simulink model "xy_graph"  (R2022a)
settings: Solver=VariableStepAuto  StartTime=0.0  StopTime=20  RelTol=1e-3
settings Model: Creator=Home  LastModifiedBy=Home

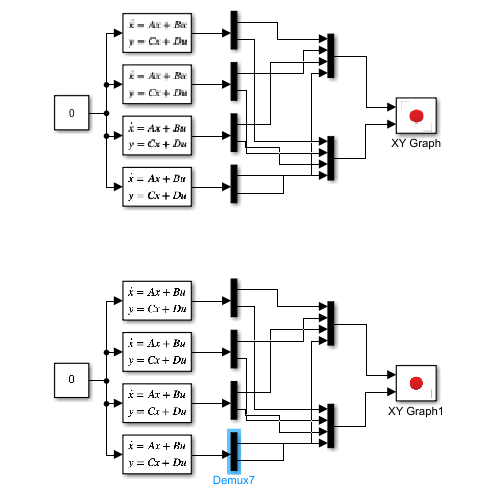
[thumbnail: Simulink's stored preview of the top-level diagram]
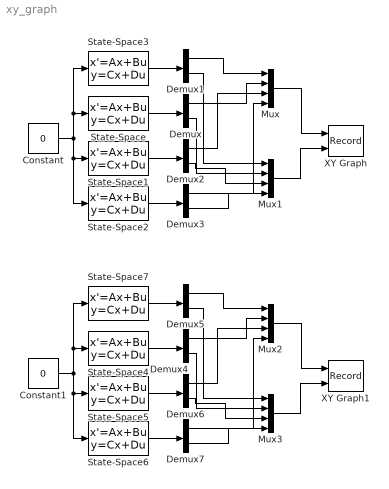
== system xy_graph ==
  Constant : Constant  Value=0
  Constant1 : Constant  Value=0
  Demux{,1..7} (8 alike) : Demux  Outputs=2
  Mux{,1..3} (4 alike) : Mux
  State-Space : StateSpace  A=[0 1; -2 1]  B=[0; 0]  C=eye(2)  D=[0; 0]  InitialCondition=[1 -1]
  State-Space1 : StateSpace  A=[0 1; -2 1]  B=[0; 0]  C=eye(2)  D=[0; 0]  InitialCondition=[-1 1]  ParameterTunability=Unconstrained
  State-Space2 : StateSpace  A=[0 1; -2 1]  B=[0; 0]  C=eye(2)  D=[0; 0]  InitialCondition=[-1 -1]  ParameterTunability=Unconstrained
  State-Space3 : StateSpace  A=[0 1; -2 1]  B=[0; 0]  C=eye(2)  D=[0; 0]  InitialCondition=[1 1]  ParameterTunability=Unconstrained
  State-Space4 : StateSpace  A=[-3 2; 1 -4]  B=[0; 0]  C=eye(2)  D=[0; 0]  InitialCondition=[500 -1000]
  State-Space5 : StateSpace  A=[-3 2; 1 -4]  B=[0; 0]  C=eye(2)  D=[0; 0]  InitialCondition=[-500 1000]  ParameterTunability=Unconstrained
  State-Space6 : StateSpace  A=[-3 2; 1 -4]  B=[0; 0]  C=eye(2)  D=[0; 0]  InitialCondition=[-500 -1000]  ParameterTunability=Unconstrained
  State-Space7 : StateSpace  A=[-3 2; 1 -4]  B=[0; 0]  C=eye(2)  D=[0; 0]  InitialCondition=[500 1000]  ParameterTunability=Unconstrained
  XY Graph : Record  FileSettingsInternal="{\"entries\":[{\"content\":{\"excelSettings\":{\"content\":{},\"type\":\"Streamout.ExcelSettings\"}},\"type\":\"Streamout.FileSettingStorage\",\"uuid\":\"1620cbbc-033e-4fe2-b11b-f0d51b19d3c6\"}],\"packageUris\":[\"http://schema.mathworks.com/mf0/streamout_blocks/R2020a\"],\"version\":\"1.0\"}"  Layout=[1 1]  SignalsInternal="{\"entries\":[{\"content\":{\"signals\":[{\"content\":{\"blockPath\":[\"xy_graph/XY Graph\"],\"channel\":[],\"dimensions\":[4],\"domain\":\"xy_graph/XY Graph\",\"hasChildren\":true,\"lineColor\":\"#edb120\",\"plots\":[],\"port\":1,\"sid\":[\"\"],\"signalID\":1160,\"signalName\":\"Mux\"},\"type\":\"RecordBlkView.Signal\",\"uuid\":\"24731fe2-5eeb-46e2-9522-8e4ef2046298\"},{\"content\":{\"blockPath\":[\"xy_graph/XY Graph\"],\"channel\":[1],\"dimensions\":[4],\"domain\":\"xy_graph/XY Graph\",\"lineColor\":\"#139fff\",\"parentID\":1160,\"plots\":[1],\"port\":1,\"sid\":[\"\"],\"signalID\":1161,\"signalName\":\"Mux\"},\"type\":\"RecordBlkView.Signal\",\"uuid\":\"67ca6b0b-c82a-407b-9284-4bd69131f7ea\"},{\"content\":{\"blockPath\":[\"xy_graph/XY Graph\"],\"channel\":[],\"dimensions\":[4],\"domain\":\"xy_graph/XY Graph\",\"hasChildren\":true,\"lineColor\":\"#77ac30\",\"plots\":[],\"port\":2,\"sid\":[\"\"],\"signalID\":1165,\"signalName\":\"Mux1\"},\"type\":\"RecordBlkView.Signal\",\"uuid\":\"273c0b79-0516-42a1-b449-bf05efc436ae\"},{\"content\":{\"blockPath\":[\"xy_graph/XY Graph\"],\"channel\":[1],\"dimensions\":[4],\"domain\":\"xy_graph/XY Graph\",\"lineColor\":\"#b746ff\",\"parentID\":1165,\"plots\":[1],\"port\":2,\"sid\":[\"\"],\"signalID\":1166,\"signalName\":\"Mux1\"},\"type\":\"RecordBlkView.Signal\",\"uuid\":\"56d8e83f-c520-44f4-8c35-4e371990f6b9\"},{\"content\":{\"blockPath\":[\"xy_graph/XY Graph\"],\"channel\":[2],\"dimensions\":[4],\"domain\":\"xy_graph/XY Graph\",\"lineColor\":\"#64d413\",\"parentID\":1160,\"plots\":[1],\"port\":1,\"sid\":[\"\"],\"signalID\":1180,\"signalName\":\"Mux\"},\"type\":\"RecordBlkView.Signal\",\"uuid\":\"527b7954-8048-4bae-9c72-ca187d897607\"},{\"content\":{\"blockPath\":[\"xy_graph/XY Graph\"],\"channel\":[3],\"dimensions\":[4],\"domain\":\"xy_graph/XY Graph\",\"lineColor\":\"#ff13a6\",\"parentID\":1160,\"plots\":[1],\"port\":1,\"sid\":[\"\"],\"signalID\":1181,\"signalName\":\"Mux\"},\"type\":\"RecordBlkView.Signal\",\"uuid\":\"88895bde-14ff-4988-9de3-88a08c4df239\"},{\"content\":{\"blockPath\":[\"xy_graph/XY Graph\"],\"channel\":[4],\"dimensions\":[4],\"domain\":\"xy_graph/XY Graph\",\"lineColor\":\"#fe330a\",\"parentID\":1160,\"plots\":[1],\"port\":1,\"sid\":[\"\"],\"signalID\":1182,\"signalName\":\"Mux\"},\"type\":\"RecordBlkView.Signal\",\"uuid\":\"b99bfa31-054d-46ce-93bd-0866448dc733\"},{\"content\":{\"blockPath\":[\"xy_graph/XY Graph\"],\"channel\":[2],\"dimensions\":[4],\"domain\":\"xy_graph/XY Graph\",\"lineColor\":\"#22b573\",\"parentID\":1165,\"plots\":[1],\"port\":2,\"sid\":[\"\"],\"signalID\":1183,\"signalName\":\"Mux1\"},\"type\":\"RecordBlkView.Signal\",\"uuid\":\"7f3c33f5-9ec2-4f34-b33e-4a0e5e9e8405\"},{\"content\":{\"blockPath\":[\"xy_graph/XY Graph\"],\"channel\":[3],\"dimensions\":[4],\"domain\":\"xy_graph/XY Graph\",\"lineColor\":\"#0072bd\",\"parentID\":1165,\"plots\":[1],\"port\":2,\"sid\":[\"\"],\"signalID\":1184,\"signalName\":\"Mux1\"},\"type\":\"RecordBlkView.Signal\",\"uuid\":\"b1473734-461a-42dd-896c-7caac445258d\"},{\"content\":{\"blockPath\":[\"xy_graph/XY Graph\"],\"channel\":[4],\"dimensions\":[4],\"domain\":\"xy_graph/XY Graph\",\"lineColor\":\"#d95319\",\"parentID\":1165,\"plots\":[1],\"port\":2,\"sid\":[\"\"],\"signalID\":1185,\"signalName\":\"Mux1\"},\"type\":\"RecordBlkView.Signal\",\"uuid\":\"044ac694-07e2-40e9-8c24-0635b6094aa9\"}]},\"type\":\"RecordBlkView.InputSignals\",\"uuid\":\"fb853018-507c-4a33-8839-1e66abb60dcd\"}],\"packageUris\":[\"http://schema.mathworks.com/mf0/streamout_blocks/R2020a\"],\"version\":\"1.0\"}"  VisualizationBindings="{\"xyplotplugin\":{\"info\":[{\"series\":[{\"bindingParametersList\":[{\"parameter\":\"X-Axis\",\"signalID\":1161,\"signalName\":\"Mux(1)\"},{\"parameter\":\"Y-Axis\",\"signalID\":1166,\"signalName\":\"Mux1(1)\"}],\"seriesID\":1003},{\"bindingParametersList\":[{\"parameter\":\"X-Axis\",\"signalID\":1180,\"signalName\":\"Mux(2)\"},{\"parameter\":\"Y-Axis\",\"signalID\":1183,\"signalName\":\"Mux1(2)\"}],\"seriesID\":908},{\"bindingParametersList\":[{\"parameter\":\"X-Axis\",\"signalID\":1181,\"signalName\":\"Mux(3)\"},{\"parameter\":\"Y-Axis\",\"signalID\":1184,\"signalName\":\"Mux1(3)\"}],\"seriesID\":917},{\"bindingParametersList\":[{\"parameter\":\"X-Axis\",\"signalID\":1182,\"signalName\":\"Mux(4)\"},{\"parameter\":\"Y-Axis\",\"signalID\":1185,\"signalName\":\"Mux1(4)\"}],\"seriesID\":762}],\"subplotID\":1}]}}"  CompatibilityTag=XY
  XY Graph1 : Record  FileSettingsInternal="{\"entries\":[{\"content\":{\"excelSettings\":{\"content\":{},\"type\":\"Streamout.ExcelSettings\"}},\"type\":\"Streamout.FileSettingStorage\",\"uuid\":\"14b4cfe2-687b-4cc5-8bba-4bb3a5f8f04c\"}],\"packageUris\":[\"http://schema.mathworks.com/mf0/streamout_blocks/R2020a\"],\"version\":\"1.0\"}"  Layout=[1 1]  SignalsInternal="{\"entries\":[{\"content\":{\"signals\":[{\"content\":{\"blockPath\":[\"xy_graph/XY Graph1\"],\"channel\":[],\"dimensions\":[4],\"domain\":\"xy_graph/XY Graph1\",\"hasChildren\":true,\"lineColor\":\"#a2142f\",\"plots\":[],\"port\":1,\"sid\":[\"\"],\"signalID\":1170,\"signalName\":\"Mux2\"},\"type\":\"RecordBlkView.Signal\",\"uuid\":\"c4bd5d30-0501-47c8-9430-780dbd134563\"},{\"content\":{\"blockPath\":[\"xy_graph/XY Graph1\"],\"channel\":[1],\"dimensions\":[4],\"domain\":\"xy_graph/XY Graph1\",\"lineColor\":\"#139fff\",\"parentID\":1170,\"plots\":[1],\"port\":1,\"sid\":[\"\"],\"signalID\":1171,\"signalName\":\"Mux2\"},\"type\":\"RecordBlkView.Signal\",\"uuid\":\"53ce3eea-74fd-400a-80a9-ce11cceb66e3\"},{\"content\":{\"blockPath\":[\"xy_graph/XY Graph1\"],\"channel\":[],\"dimensions\":[4],\"domain\":\"xy_graph/XY Graph1\",\"hasChildren\":true,\"lineColor\":\"#ff6929\",\"plots\":[],\"port\":2,\"sid\":[\"\"],\"signalID\":1175,\"signalName\":\"Mux3\"},\"type\":\"RecordBlkView.Signal\",\"uuid\":\"d0be590c-aa50-459b-9930-31eb964dbcd6\"},{\"content\":{\"blockPath\":[\"xy_graph/XY Graph1\"],\"channel\":[1],\"dimensions\":[4],\"domain\":\"xy_graph/XY Graph1\",\"lineColor\":\"#b746ff\",\"parentID\":1175,\"plots\":[1],\"port\":2,\"sid\":[\"\"],\"signalID\":1176,\"signalName\":\"Mux3\"},\"type\":\"RecordBlkView.Signal\",\"uuid\":\"e2dc7741-9486-4c53-8038-f7524e7cc87c\"},{\"content\":{\"blockPath\":[\"xy_graph/XY Graph1\"],\"channel\":[2],\"dimensions\":[4],\"domain\":\"xy_graph/XY Graph1\",\"lineColor\":\"#64d413\",\"parentID\":1170,\"plots\":[1],\"port\":1,\"sid\":[\"\"],\"signalID\":1186,\"signalName\":\"Mux2\"},\"type\":\"RecordBlkView.Signal\",\"uuid\":\"9c9cff46-c965-4e97-80cb-7be04a75b3bd\"},{\"content\":{\"blockPath\":[\"xy_graph/XY Graph1\"],\"channel\":[3],\"dimensions\":[4],\"domain\":\"xy_graph/XY Graph1\",\"lineColor\":\"#ff13a6\",\"parentID\":1170,\"plots\":[1],\"port\":1,\"sid\":[\"\"],\"signalID\":1187,\"signalName\":\"Mux2\"},\"type\":\"RecordBlkView.Signal\",\"uuid\":\"14e05be8-f402-434d-b11b-945623433030\"},{\"content\":{\"blockPath\":[\"xy_graph/XY Graph1\"],\"channel\":[4],\"dimensions\":[4],\"domain\":\"xy_graph/XY Graph1\",\"lineColor\":\"#fe330a\",\"parentID\":1170,\"plots\":[1],\"port\":1,\"sid\":[\"\"],\"signalID\":1188,\"signalName\":\"Mux2\"},\"type\":\"RecordBlkView.Signal\",\"uuid\":\"51e92ddc-1328-4d24-8d38-5f4391dd10c3\"},{\"content\":{\"blockPath\":[\"xy_graph/XY Graph1\"],\"channel\":[2],\"dimensions\":[4],\"domain\":\"xy_graph/XY Graph1\",\"lineColor\":\"#22b573\",\"parentID\":1175,\"plots\":[1],\"port\":2,\"sid\":[\"\"],\"signalID\":1189,\"signalName\":\"Mux3\"},\"type\":\"RecordBlkView.Signal\",\"uuid\":\"6abbcd08-1459-40ca-856f-07b3b545ec3b\"},{\"content\":{\"blockPath\":[\"xy_graph/XY Graph1\"],\"channel\":[3],\"dimensions\":[4],\"domain\":\"xy_graph/XY Graph1\",\"lineColor\":\"#0072bd\",\"parentID\":1175,\"plots\":[1],\"port\":2,\"sid\":[\"\"],\"signalID\":1190,\"signalName\":\"Mux3\"},\"type\":\"RecordBlkView.Signal\",\"uuid\":\"474a5ab5-9738-4c4a-8e36-9efeb30e4c06\"},{\"content\":{\"blockPath\":[\"xy_graph/XY Graph1\"],\"channel\":[4],\"dimensions\":[4],\"domain\":\"xy_graph/XY Graph1\",\"lineColor\":\"#d95319\",\"parentID\":1175,\"plots\":[1],\"port\":2,\"sid\":[\"\"],\"signalID\":1191,\"signalName\":\"Mux3\"},\"type\":\"RecordBlkView.Signal\",\"uuid\":\"6fb3bfb3-fd05-446e-94dc-7b800bd07288\"}]},\"type\":\"RecordBlkView.InputSignals\",\"uuid\":\"cc4b9596-2de2-40f4-a5ef-2b0ca2047e51\"}],\"packageUris\":[\"http://schema.mathworks.com/mf0/streamout_blocks/R2020a\"],\"version\":\"1.0\"}"  VisualizationBindings="{\"xyplotplugin\":{\"info\":[{\"series\":[{\"bindingParametersList\":[{\"parameter\":\"X-Axis\",\"signalID\":1171,\"signalName\":\"Mux2(1)\"},{\"parameter\":\"Y-Axis\",\"signalID\":1176,\"signalName\":\"Mux3(1)\"}],\"seriesID\":48271},{\"bindingParametersList\":[{\"parameter\":\"X-Axis\",\"signalID\":1186,\"signalName\":\"Mux2(2)\"},{\"parameter\":\"Y-Axis\",\"signalID\":1189,\"signalName\":\"Mux3(2)\"}],\"seriesID\":39449},{\"bindingParametersList\":[{\"parameter\":\"X-Axis\",\"signalID\":1187,\"signalName\":\"Mux2(3)\"},{\"parameter\":\"Y-Axis\",\"signalID\":1190,\"signalName\":\"Mux3(3)\"}],\"seriesID\":6787},{\"bindingParametersList\":[{\"parameter\":\"X-Axis\",\"signalID\":1188,\"signalName\":\"Mux2(4)\"},{\"parameter\":\"Y-Axis\",\"signalID\":1191,\"signalName\":\"Mux3(4)\"}],\"seriesID\":5061}],\"subplotID\":1}]}}"  CompatibilityTag=XY
  wires:
  State-Space/1 -> Demux/1
  Constant/1 -> State-Space2/1, State-Space1/1, State-Space3/1, State-Space/1
  State-Space3/1 -> Demux1/1
  State-Space1/1 -> Demux2/1
  State-Space2/1 -> Demux3/1
  Demux1/1 -> Mux/1
  Demux/1 -> Mux/2
  Demux2/1 -> Mux/3
  Demux3/1 -> Mux/4
  Mux/1 -> XY Graph/1
  Demux1/2 -> Mux1/1
  Demux/2 -> Mux1/2
  Demux2/2 -> Mux1/3
  Demux3/2 -> Mux1/4
  Mux1/1 -> XY Graph/2
  Demux4/2 -> Mux3/2
  Demux5/2 -> Mux3/1
  Demux6/2 -> Mux3/3
  Demux7/2 -> Mux3/4
  Demux6/1 -> Mux2/3
  Mux2/1 -> XY Graph1/1
  State-Space5/1 -> Demux6/1
  Demux4/1 -> Mux2/2
  Mux3/1 -> XY Graph1/2
  Demux7/1 -> Mux2/4
  State-Space6/1 -> Demux7/1
  State-Space7/1 -> Demux5/1
  Demux5/1 -> Mux2/1
  Constant1/1 -> State-Space6/1, State-Space5/1, State-Space7/1, State-Space4/1
  State-Space4/1 -> Demux4/1
